simulink model "fil"  (R2021a)
settings: Solver=VariableStepAuto  StartTime=0.0  StopTime=10.0  RelTol=1e-3
libraries: dspsrcs4 x2, dsparch4 x1
settings Model: Creator=kunch  LastModifiedBy=kunch

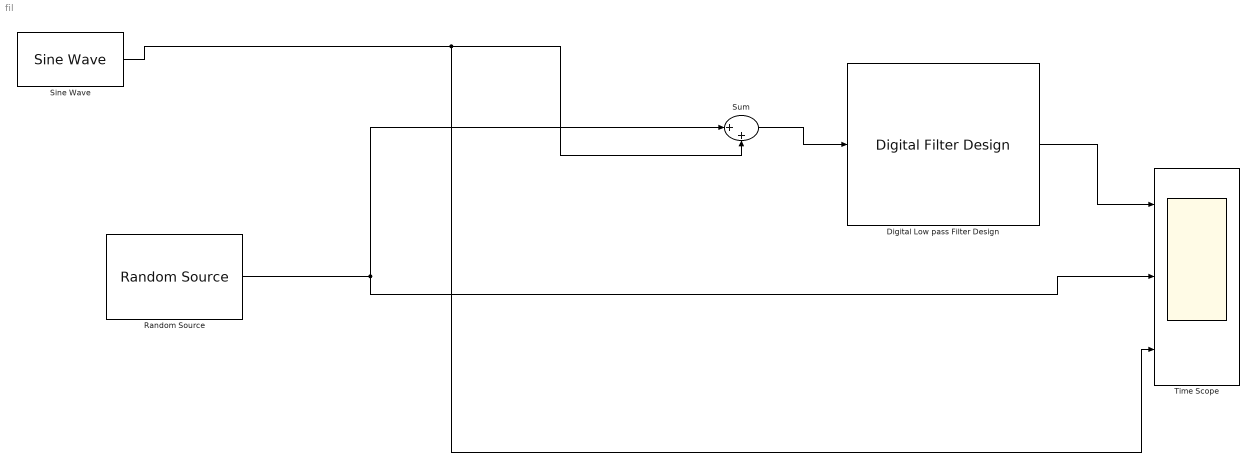
== system fil ==
  Digital Low pass Filter Design : dsparch4/Digital Filter Design  mwdsp_browser_bugfix_var=off
  Random Source : dspsrcs4/Random Source  SrcType=Uniform  NormMethod=Ziggurat  CltLength=12  MinVal=0  MaxVal=4  MeanVal=0  VarVal=1  RepMode=Not repeatable  rawSeed=1  IsInherit=off  SampMode=Discrete  SampTime=1/1000  SampFrame=5  DataType=Double  OutComplex=Real  OutputFrames=off
  Sine Wave : dspsrcs4/Sine Wave  Amplitude=1  Frequency=100  Phase=0  SampleMode=Discrete  OutComplex=Real  CompMethod=Trigonometric fcn  TableSize=Speed  SampleTime=1/1000  SamplesPerFrame=1  ResetState=Restart at time zero  OutputFrames=off  dataType=double  wordLen=16  udDataType=sfix(16)  fracBitsMode=Best precision  numFracBits=15  OutDataTypeStr=double  LastOutDataTypeStr=double
  Sum : Sum  Inputs=|++
  Time Scope : Scope  NumInputPorts=3
  wires:
  Random Source/1 -> Time Scope/2, Sum/1
  Sum/1 -> Digital Low pass Filter Design/1
  Digital Low pass Filter Design/1 -> Time Scope/1
  Sine Wave/1 -> Time Scope/3, Sum/2
